simulink library "Lib_PF_XformerAAC_TMATS"  (R2017a)
settings: Solver=ode45  StartTime=0.0  StopTime=10.0  RelTol=1e-3  EnableMultiTasking=on
Description:
  | Thomas Modules
settings Model: Creator=jwchapm2  LastModifiedBy=glthoma1
settings DataIOCC: LimitDataPoints=on  SaveFormat=Array
settings OptimizationCC: ExpressionDepthLimit=2147483647  LifeSpan=inf
settings DebuggingCC: UnderspecifiedInitializationDetection=Classic  MergeDetectMultiDrivingBlocksExec=none  SolverPrmCheckMsg=warning  StateNameClashWarn=warning  SFUnexpectedBacktrackingDiag=warning  SFNoUnconditionalDefaultTransitionDiag=warning  SFExecutionAtInitializationDiag=none
settings HardwareCC: ProdBitPerPointer=32  ProdBitPerSizeT=32  ProdBitPerPtrDiffT=32  ProdLargestAtomicFloat=None  ProdIntDivRoundTo=Undefined  ProdEndianess=Unspecified  ProdWordSize=32  ProdHWDeviceType=32-bit Generic
settings ModelReferenceCC: PropagateSignalLabelsOutOfModel=off
settings GRTTargetCC: TargetLangStandard=C89/C90 (ANSI)  GeneratePreprocessorConditionals=Disable all
settings ConfigComp: CovMetricSettings=dw  CovHtmlReporting=on  CovSaveCumulativeToWorkspaceVar=on  CovSaveSingleToWorkspaceVar=on  CovExternalEMLEnable=off

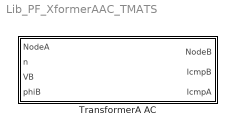
== system Lib_PF_XformerAAC_TMATS ==
  TransformerA AC : Subsystem  mask{R_M=1, X_M=0, alpha_M=0, b_M=1}
      mask prompts: R_M "R_M - Resistance"; X_M "X_M - Reactance"; alpha_M "alpha_M - controlled phase shift"; b_M "b_M - system voltage ratio"
      mask Display:
      | fprintf('c_bar : 1\nZ = R + jX\n %g + j%g\n controlled phase shift:%g\n system voltage ratio:%g',R_M, X_M,alpha_M,b_M)
      | port_label('input',1,'VA')
      | port_label('input',2,'n')
      | port_label('input',3,'VBg')
      | port_label('input',4,'phiBg')
      | port_label('output',1,'VB')
      | port_label('output',2,'IcB')
      | port_label('output',3,'IcA')

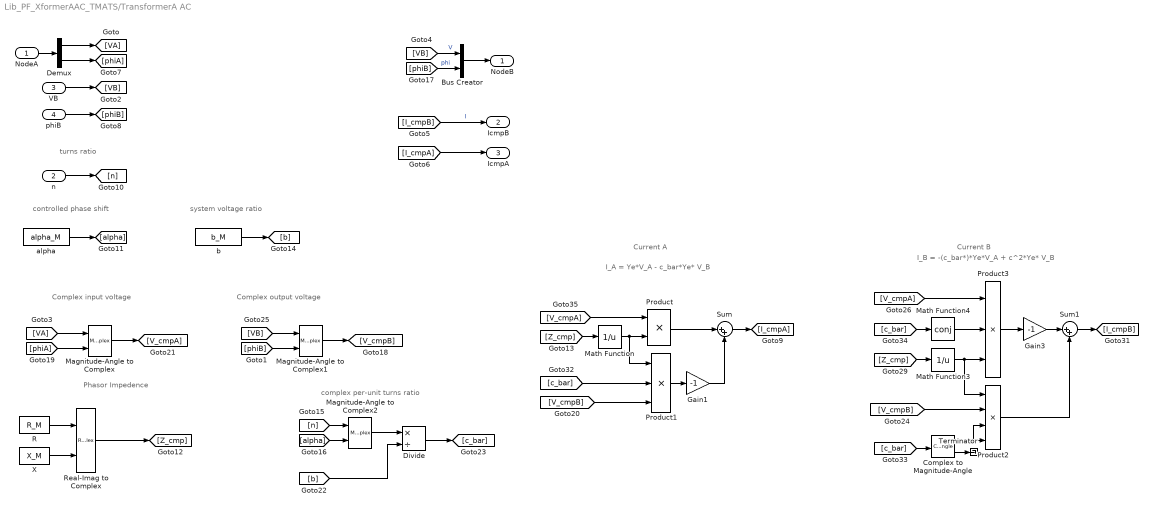
== system Lib_PF_XformerAAC_TMATS/TransformerA AC ==
  note: I_A = Ye*V_A - c_bar*Ye* V_B
  note: Complex output voltage
  note: Complex input voltage
  note: Phasor Impedence
  note: Current A
  note: turns ratio
  note: controlled phase shift
  note: system voltage ratio
  note: complex per-unit turns ratio
  note: Current B
  note: I_B = -(c_bar*)*Ye*V_A + c^2*Ye* V_B
  NodeA : Inport
  n : Inport  Port=2
  VB : Inport  Port=3
  phiB : Inport  Port=4
  Bus Creator : BusCreator  Inputs=2
  Complex to Magnitude-Angle : ComplexToMagnitudeAngle
  Demux : Demux  Outputs=2
  Divide : Product  Inputs=*/
  Gain1 : Gain  Gain=-1
  Gain3 : Gain  Gain=-1
  Magnitude-Angle to Complex : MagnitudeAngleToComplex
  Magnitude-Angle to Complex1 : MagnitudeAngleToComplex
  Magnitude-Angle to Complex2 : MagnitudeAngleToComplex
  Math Function : Math  Operator=reciprocal  SaturateOnIntegerOverflow=on
  Math Function3 : Math  Operator=reciprocal  SaturateOnIntegerOverflow=on
  Math Function4 : Math  Operator=conj  SaturateOnIntegerOverflow=on
  Product : Product
  Product1 : Product  Inputs=3
  Product2 : Product  Inputs=4
  Product3 : Product  Inputs=3
  R : Constant  Value=R_M
  Real-Imag to Complex : RealImagToComplex
  Sum : Sum  Inputs=|++
  Sum1 : Sum  Inputs=|++
  Terminator : Terminator
  X : Constant  Value=X_M
  alpha : Constant  Value=alpha_M
  b : Constant  Value=b_M
  NodeB : Outport
  IcmpB : Outport  Port=2
  IcmpA : Outport  Port=3
  wires:
  Demux/1 -> [VA]
  [phiB] -> Bus Creator/2  "phi"
  [I_cmpB] -> IcmpB/1  "I"
  phiB/1 -> [phiB]
  Demux/2 -> [phiA]
  NodeA/1 -> Demux/1
  VB/1 -> [VB]
  [VB] -> Bus Creator/1  "V"
  Bus Creator/1 -> NodeB/1
  [VA] -> Magnitude-Angle to Complex/1
  [phiA] -> Magnitude-Angle to Complex/2
  Magnitude-Angle to Complex/1 -> [V_cmpA]
  [VB] -> Magnitude-Angle to Complex1/1
  Magnitude-Angle to Complex1/1 -> [V_cmpB]
  [phiB] -> Magnitude-Angle to Complex1/2
  R/1 -> Real-Imag to Complex/1
  X/1 -> Real-Imag to Complex/2
  Real-Imag to Complex/1 -> [Z_cmp]
  [V_cmpA] -> Product/1
  [Z_cmp] -> Math Function/1
  Sum/1 -> [I_cmpA]
  Math Function/1 -> Product1/1, Product/2
  [I_cmpA] -> IcmpA/1
  n/1 -> [n]
  alpha/1 -> [alpha]
  b/1 -> [b]
  [n] -> Magnitude-Angle to Complex2/1
  [alpha] -> Magnitude-Angle to Complex2/2
  Magnitude-Angle to Complex2/1 -> Divide/1
  [b] -> Divide/2
  Divide/1 -> [c_bar]
  Product/1 -> Sum/1
  Product1/1 -> Gain1/1
  Gain1/1 -> Sum/2
  Sum1/1 -> [I_cmpB]
  Product2/1 -> Sum1/2
  [c_bar] -> Product1/2
  Gain3/1 -> Sum1/1
  [c_bar] -> Complex to Magnitude-Angle/1
  Complex to Magnitude-Angle/1 -> Product2/3, Product2/4
  Complex to Magnitude-Angle/2 -> Terminator/1
  Math Function3/1 -> Product2/1, Product3/3
  [Z_cmp] -> Math Function3/1
  [V_cmpA] -> Product3/1
  Product3/1 -> Gain3/1
  [c_bar] -> Math Function4/1
  Math Function4/1 -> Product3/2
  [V_cmpB] -> Product1/3
  [V_cmpB] -> Product2/2
